simulink model "Project_Garage_Door_Opener"  (R2020b)
settings: Solver=VariableStepAuto  StartTime=0.0  StopTime=50  RelTol=1e-3
undefined symbols (not defined in the file): sigbuilder_block
libraries: fl_lib x8, nesl_utility x3, simulink_extras x2, powerlib_meascontrol x1
settings Model: EnablePacing=on  Creator=ricar  LastModifiedBy=ricar

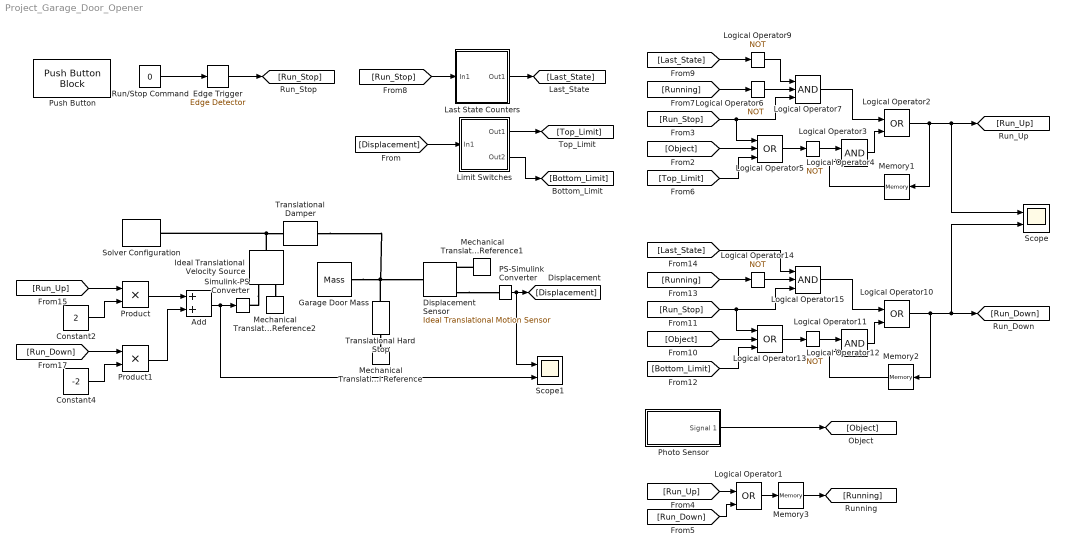
== system Project_Garage_Door_Opener ==
  Add : Sum
  Constant2 : Constant  Value=2
  Constant4 : Constant  Value=-2
  Displacement Sensor : fl_lib/Mechanical/Mechanical Sensors/Ideal Translational Motion Sensor  offset=0 m
  Edge Trigger : powerlib_meascontrol/Logic/Edge Detector  model=Rising  ic=0  Ts=-1
      settings: SourceProductBaseCode=PS
  Garage Door Mass : fl_lib/Mechanical/Translational Elements/Mass  mass=100 kg  num_ports=foundation.enum.numPorts2.one  v_specify=off  v_priority=High  v=0 m/s  v_nominal_specify=off  v_nominal_unit=m/s  v_nominal_value=1  f_specify=off  f_priority=None  f=0 N  f_nominal_specify=off  f_nominal_unit=N  f_nominal_value=1
  Ideal Translational Velocity Source : fl_lib/Mechanical/Mechanical Sources/Ideal Translational Velocity Source
  Last State Counters : Subsystem
  Limit Switches : Subsystem
  Logical Operator1 : Logic  Operator=OR  IconShape=distinctive  AllPortsSameDT=off  OutDataTypeStr=boolean
  Logical Operator10 : Logic  Operator=OR  IconShape=distinctive  AllPortsSameDT=off  OutDataTypeStr=boolean
  Logical Operator11 : Logic  IconShape=distinctive  AllPortsSameDT=off  OutDataTypeStr=boolean
  Logical Operator{4,6,9,12,14} (5 alike) : Logic  Operator=NOT  IconShape=distinctive  AllPortsSameDT=off  OutDataTypeStr=boolean
  Logical Operator13 : Logic  Operator=OR  Inputs=3  IconShape=distinctive  AllPortsSameDT=off  OutDataTypeStr=boolean
  Logical Operator15 : Logic  Inputs=3  IconShape=distinctive  AllPortsSameDT=off  OutDataTypeStr=boolean
  Logical Operator2 : Logic  Operator=OR  IconShape=distinctive  AllPortsSameDT=off  OutDataTypeStr=boolean
  Logical Operator3 : Logic  IconShape=distinctive  AllPortsSameDT=off  OutDataTypeStr=boolean
  Logical Operator5 : Logic  Operator=OR  Inputs=3  IconShape=distinctive  AllPortsSameDT=off  OutDataTypeStr=boolean
  Logical Operator7 : Logic  Inputs=3  IconShape=distinctive  AllPortsSameDT=off  OutDataTypeStr=boolean
  Mechanical Translational Reference : fl_lib/Mechanical/Translational Elements/Mechanical Translational Reference
  Mechanical Translational Reference1 : fl_lib/Mechanical/Translational Elements/Mechanical Translational Reference
  Mechanical Translational Reference2 : fl_lib/Mechanical/Translational Elements/Mechanical Translational Reference
  Memory1 : Memory
  Memory2 : Memory
  Memory3 : Memory  InheritSampleTime=on
  PS-Simulink Converter : nesl_utility/PS-Simulink Converter  PhysicalDomain=network_engine_domain  SubClassName=ps_output  LeftPortType=input  RightPortType=output  PseudoPeriodic=off  Frequencies=[]  Unit=inherit  AffineConversion=off
  Photo Sensor : Subsystem  Tag=STV Subsys  LoadFcn=sigbuilder_block('load',[273.667 100 580 400 ]);  StartFcn=sigbuilder_block('start');  StopFcn=sigbuilder_block('stop');  ClipboardFcn=sigbuilder_block('clipboard');  mask(Sigbuilder block){tuvar=[0:10]}
      mask help: Simulink:masks:SigbuilderBlock_MD
      mask init:
      | if ~strcmp(get_param(bdroot(gcbh),'SimulationStatus'),'stopped') tuvar = sigbuilder_block('maskInit'); end
      settings: CopyFcn=sigbuilder_block('copy');  DeleteFcn=sigbuilder_block('delete');  ModelCloseFcn=sigbuilder_block('modelClose');  PreSaveFcn=sigbuilder_block('preSave');  PauseFcn=sigbuilder_block('pause');  ContinueFcn=sigbuilder_block('continue');  NameChangeFcn=sigbuilder_block('namechange');  OpenFcn=sigbuilder_block('open',[273.667 100 580 400 ]);  CloseFcn=sigbuilder_block('close');
      mask Display: plot(0, 0, 100, 100,[2, 2, 32, 32, 2], [68, 8, 8, 68, 68],[32, 2], [38, 38], [32, 19, 2],[53, 60, 44], [32, 17, 17, 2],[16, 16, 31, 31]);txt = getActiveGroup(gcbh);text(2, 100, txt,'verticalAlignment', 'top');
  Product : Product
  Product1 : Product
  Push Button : PushButtonBlock  ButtonText=Push Button
  Run/Stop Command : Constant  Value=0  OutDataTypeStr=boolean
  Scope : Scope  NumInputPorts=2
  Scope1 : Scope  NumInputPorts=2
  Simulink-PS Converter : nesl_utility/Simulink-PS Converter  PhysicalDomain=network_engine_domain  SubClassName=ps_input  LeftPortType=input  RightPortType=output  PseudoPeriodic=off  Frequencies=[]  NoiseDistribution=none  NoiseParameters=[]  Unit=1  AffineConversion=off  FilteringAndDerivatives=provide  SimscapeFilterOrder=1  InputFilterTimeConstant=0.001  UdotUserProvided=0
  Solver Configuration : nesl_utility/Solver Configuration  PhysicalDomain=network_engine_domain  SubClassName=solver  LeftPortType=input  RightPortType=generic  Tones=[]  Harmonics=[]  SimulateNoise=off  Profile=off  UseLocalSampling=off  EnableSwitchedLinearOptims=on  FrequencyDomain=off  UseCCode=off  RelTol=0.001  AbsTol=1e-06  MinStep=1e-09  ToWorkspace=off  RevertToSquareIcSolve=off  NumHomotopyIterations=100  PhasorMode=off  PhasorModeNumHarmonics=1  DoDC=off  ResidualTolerance=1e-09  UseLocalSolver=on  LocalSolverChoice=NE_BACKWARD_EULER_ADVANCER  LocalSolverSampleTime=0.001  DoFixedCost=on  MaxNonlinIter=3  MaxModeIter=2  ComputeImpulses=off  ImpulseIterations=2  LinearAlgebra=auto  EquationFormulation=NE_TIME_EF  DelaysMemoryBudget=1024  AutomaticFiltering=on  FilteringTimeConstant=0.001  PartitionStorageMethod=AS_NEEDED  PartitionMemoryBudget=1024  PartitionMethod=ROBUST
  Translational Damper : fl_lib/Mechanical/Translational Elements/Translational Damper  D=1000 N/(m/s)  v_specify=off  v_priority=None  v=0 m/s  v_nominal_specify=off  v_nominal_unit=m/s  v_nominal_value=1  f_specify=off  f_priority=None  f=0 N  f_nominal_specify=off  f_nominal_unit=N  f_nominal_value=1
  Translational Hard Stop : fl_lib/Mechanical/Translational Elements/Translational Hard Stop  upper_bnd=10 m  lower_bnd=0 m  stiff_up=1e6 N/m  stiff_low=1e6 N/m  D_up=150 N/(m/s)  D_low=150 N/(m/s)  model=simscape.enum.hardstop.smooth  transition=1 m  v_specify=off  v_priority=None  v=0 m/s  v_nominal_specify=off  v_nominal_unit=m/s  v_nominal_value=1  f_specify=off  f_priority=None  f=0 N  f_nominal_specify=off  f_nominal_unit=N  f_nominal_value=1  x_specify=off  x_priority=High  x=0 m  x_nominal_specify=off  x_nominal_unit=m  x_nominal_value=1
  wires:
  Photo Sensor/1(Signal 1) -> [Object]
  Logical Operator3/1 -> Logical Operator2/2
  Logical Operator4/1 -> Logical Operator3/1
  Logical Operator2/1 -> Memory1/1, Scope/1, [Run_Up]
  [Run_Stop] -> Logical Operator7/3, Logical Operator5/1
  [Run_Up] -> Logical Operator1/1
  [Run_Down] -> Logical Operator1/2
  Logical Operator5/1 -> Logical Operator4/1
  [Object] -> Logical Operator5/2
  [Running] -> Logical Operator6/1
  Logical Operator7/1 -> Logical Operator2/1
  Logical Operator6/1 -> Logical Operator7/2
  [Last_State] -> Logical Operator9/1
  Logical Operator9/1 -> Logical Operator7/1
  Logical Operator11/1 -> Logical Operator10/2
  Logical Operator15/1 -> Logical Operator10/1
  [Run_Stop] -> Logical Operator15/3, Logical Operator13/1
  [Last_State] -> Logical Operator15/1
  Logical Operator13/1 -> Logical Operator12/1
  [Running] -> Logical Operator14/1
  [Object] -> Logical Operator13/2
  Logical Operator10/1 -> Memory2/1, Scope/2, [Run_Down]
  Logical Operator12/1 -> Logical Operator11/1
  Logical Operator14/1 -> Logical Operator15/2
  Memory1/1 -> Logical Operator3/2
  Memory2/1 -> Logical Operator11/2
  Logical Operator1/1 -> Memory3/1
  Memory3/1 -> [Running]
  Run/Stop Command/1 -> Edge Trigger/1
  Edge Trigger/1 -> [Run_Stop]
  Add/1 -> Scope1/2, Simulink-PS Converter/1
  [Run_Up] -> Product/1
  PS-Simulink Converter/1 -> Scope1/1, [Displacement]
  Constant2/1 -> Product/2
  Constant4/1 -> Product1/2
  [Run_Down] -> Product1/1
  Product/1 -> Add/1
  Product1/1 -> Add/2
  [Top_Limit] -> Logical Operator5/3
  [Bottom_Limit] -> Logical Operator13/3
  [Run_Stop] -> Last State Counters/1(In1)
  Last State Counters/1(Out1) -> [Last_State]
  [Displacement] -> Limit Switches/1(In1)
  Limit Switches/1(Out1) -> [Top_Limit]
  Limit Switches/2(Out2) -> [Bottom_Limit]
  connections:
  Garage Door Mass/LConn1 -- Translational Damper/RConn1 -- Translational Hard Stop/LConn1 -- Displacement Sensor/LConn1
  Displacement Sensor/RConn3 -- PS-Simulink Converter/LConn1
  Ideal Translational Velocity Source/RConn1 -- Simulink-PS Converter/RConn1
  Translational Hard Stop/RConn1 -- Mechanical Translational Reference/LConn1
  Ideal Translational Velocity Source/RConn2 -- Mechanical Translational Reference2/LConn1
  Ideal Translational Velocity Source/LConn1 -- Solver Configuration/RConn1 -- Translational Damper/LConn1
  Mechanical Translational Reference1/LConn1 -- Displacement Sensor/RConn1

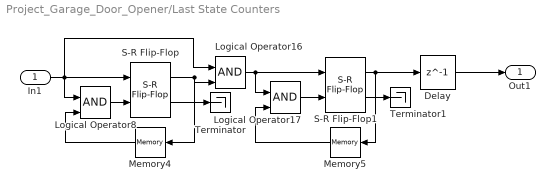
== system Project_Garage_Door_Opener/Last State Counters ==
  In1 : Inport
  Delay : Delay  DelayLength=1  InitialCondition=0
  Logical Operator16 : Logic  IconShape=distinctive  AllPortsSameDT=off  OutDataTypeStr=boolean
  Logical Operator17 : Logic  IconShape=distinctive  AllPortsSameDT=off  OutDataTypeStr=boolean
  Logical Operator8 : Logic  IconShape=distinctive  AllPortsSameDT=off  OutDataTypeStr=boolean
  Memory4 : Memory  InheritSampleTime=on
  Memory5 : Memory  InheritSampleTime=on
  S-R Flip-Flop : simulink_extras/Flip Flops/S-R Flip-Flop  initial_condition=0
  S-R Flip-Flop1 : simulink_extras/Flip Flops/S-R Flip-Flop  initial_condition=0
  Terminator : Terminator
  Terminator1 : Terminator
  Out1 : Outport
  wires:
  Logical Operator16/1 -> Logical Operator17/1, S-R Flip-Flop1/1
  S-R Flip-Flop/2 -> Terminator/1
  In1/1 -> Logical Operator16/1, S-R Flip-Flop/1, Logical Operator8/1
  Logical Operator8/1 -> S-R Flip-Flop/2
  S-R Flip-Flop1/2 -> Terminator1/1
  Memory4/1 -> Logical Operator8/2
  Memory5/1 -> Logical Operator17/2
  Delay/1 -> Out1/1
  S-R Flip-Flop1/1 -> Delay/1, Memory5/1
  S-R Flip-Flop/1 -> Logical Operator16/2, Memory4/1
  Logical Operator17/1 -> S-R Flip-Flop1/2

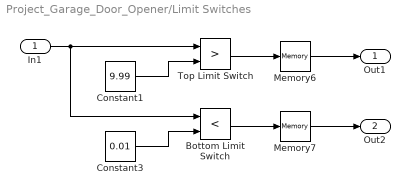
== system Project_Garage_Door_Opener/Limit Switches ==
  In1 : Inport
  Bottom Limit Switch : RelationalOperator  Operator=<  OutDataTypeStr=boolean  RndMeth=Simplest
  Constant1 : Constant  Value=9.99
  Constant3 : Constant  Value=0.01
  Memory6 : Memory  InheritSampleTime=on
  Memory7 : Memory  InheritSampleTime=on
  Top Limit Switch : RelationalOperator  Operator=>  OutDataTypeStr=boolean  RndMeth=Simplest
  Out1 : Outport
  Out2 : Outport  Port=2
  wires:
  Constant1/1 -> Top Limit Switch/2
  In1/1 -> Bottom Limit Switch/1, Top Limit Switch/1
  Bottom Limit Switch/1 -> Memory7/1
  Memory6/1 -> Out1/1
  Top Limit Switch/1 -> Memory6/1
  Constant3/1 -> Bottom Limit Switch/2
  Memory7/1 -> Out2/1

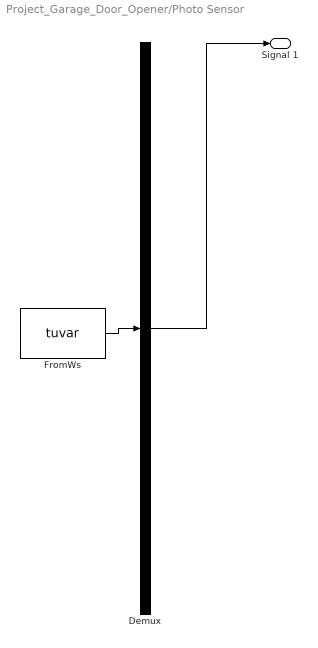
== system Project_Garage_Door_Opener/Photo Sensor ==
  Demux : Demux  Tag=STV Demux  Outputs=1
      settings: DisplayOption=none
  FromWs : FromWorkspace  Tag=STV FromWs  VariableName=tuvar
      SigBuilderData=|
      | common.afterFinalStr = 'Extrapolate'
      | common.sampleTime = '0'
      | dataSet.timeRange = [0 50]
      | dataSet.name = 'Group 1'
      | sbobj.Groups.Name = 'Group 1'
      | sbobj.Groups.Signals.Name = 'Signal 1'
      | sbobj.Groups.Signals.XData = [0 5 5 40 40 50]
      | sbobj.Groups.Signals.YData = [0 0 1 1 0 0]
      | sbobj.Groups.TimeRange = [0 50]
  Signal 1 : Outport  Tag=STV Outport
  wires:
  Demux/1 -> Signal 1/1
  FromWs/1 -> Demux/1
